simulink model "UDPrcv_Mac"  (R2014b)
settings: Solver=FixedStepDiscrete  StartTime=0.0  StopTime=inf  FixedStep=0.025  RelTol=1e-3
InitFcn:
  | Ts=0.025;
libraries: simulink x2, dspnetwork x1
settings Model: Creator=FranR  LastModifiedBy=FranR

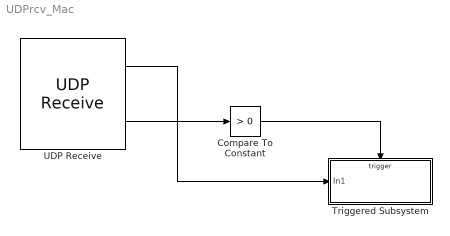
== system UDPrcv_Mac ==
  Compare To Constant : simulink/Logic and Bit Operations/Compare To Constant  relop=>  const=0  OutDataTypeStr=boolean
  Triggered Subsystem : Subsystem  TreatAsAtomicUnit=on
  UDP Receive : dspnetwork/UDP Receive  localURL='0.0.0.0'  localPort=7500  remoteURL='192.168.7.2'  remotePort=-1  recvBufferSize=1024  dims=6  signalDatatype=uint8  isVarSize=off  showBlockingTime=off  blockingTime=0  sampletime=0.025
  wires:
  UDP Receive/2 -> Compare To Constant/1
  Compare To Constant/1 -> Triggered Subsystem/Trigger
  UDP Receive/1 -> Triggered Subsystem/1(In1)

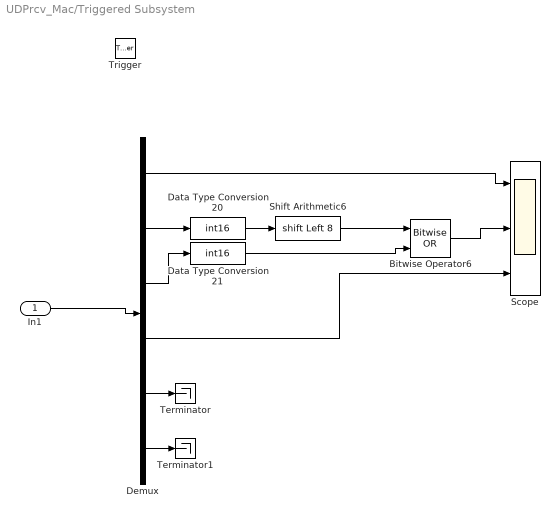
== system UDPrcv_Mac/Triggered Subsystem ==
  In1 : Inport
  Trigger : TriggerPort
  Bitwise Operator6 : simulink/Logic and Bit Operations/Bitwise Operator  logicop=OR  UseBitMask=off  NumInputPorts=2  BitMask=bin2dec('11011001')  BitMaskRealWorld=Stored Integer
  Data Type Conversion20 : DataTypeConversion  OutDataTypeStr=int16
  Data Type Conversion21 : DataTypeConversion  OutDataTypeStr=int16
  Demux : Demux  Outputs=6
  Scope : Scope  NumInputPorts=3
      settings: TimeRange=10000  YMin=99~0~0  YMax=101~361~300
  Shift Arithmetic6 : ArithShift  BitShiftNumber=8  BitShiftDirection=Left
  Terminator : Terminator
  Terminator1 : Terminator
  wires:
  In1/1 -> Demux/1
  Demux/1 -> Scope/1
  Data Type Conversion21/1 -> Bitwise Operator6/2
  Shift Arithmetic6/1 -> Bitwise Operator6/1
  Data Type Conversion20/1 -> Shift Arithmetic6/1
  Demux/2 -> Data Type Conversion20/1
  Demux/3 -> Data Type Conversion21/1
  Demux/4 -> Scope/3
  Bitwise Operator6/1 -> Scope/2
  Demux/5 -> Terminator/1
  Demux/6 -> Terminator1/1
